simulink model "teste"  (R2020b)
settings: Solver=FixedStepAuto  StartTime=0.0  StopTime=10.0  RelTol=1e-3
settings Model: Creator=amarc  LastModifiedBy=amarc

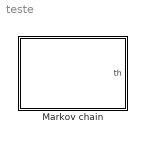
== system teste ==
  Markov chain : Subsystem

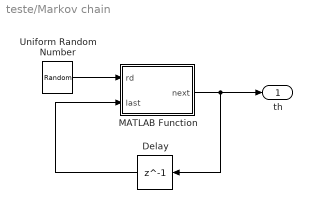
== system teste/Markov chain ==
  Delay : Delay  DelayLength=1
  MATLAB Function : MATLAB Function  TreatAsAtomicUnit=on
  Uniform Random Number : UniformRandomNumber  Minimum=0
  th : Outport
  wires:
  MATLAB Function/1(next) -> th/1, Delay/1
  Delay/1 -> MATLAB Function/2(last)
  Uniform Random Number/1 -> MATLAB Function/1(rd)

== matlab function teste/Markov chain/MATLAB Function ==
  data: rd input; next output; last input
function next = fcn(rd,last)

mu = [0.7 0.2 0.1];
P = [0.7 0.2 0.1;0.3 0.7 0;0.1 0.5 0.4];
N= 3;
aux_next = 0;

if last == 0
    mu_aux = [0 cumsum(mu)];
    for i = 1:N
        if (mu_aux(i) <  rd)&&(rd <= mu_aux(i+1)) 
            aux_next = i;
        end
    end
else
    mu_aux = [0 cumsum(P(last,:))];
    for i = 1:N
        if (mu_aux(i) <  rd)&&(rd <= mu_aux(i+1)) 
            aux_next = i;
        end
    end
end
next = aux_next;
